simulink model "c221127_FCEV_SLMP_SQP"  (R2022b)
settings: Solver=FixedStepAuto  StartTime=0.0  StopTime=DrvCycLen  FixedStep=1  RelTol=1e-3
values from neighbouring files (symbols this model uses):
  AccThrshd = 1    [Config_c221112.m]    (also in Config_c221127.m; Config_c221218.m; Config_c230117.m; Config_c230321.m)
  AlphaRampFactor = 8    [Config_c221112.m]    (also in Config_c221127.m; Config_c221218.m; Config_c230117.m; Config_c230321.m)
  Bat_eff_chg_average = 0.969    [FCEV_original_data.mat]
  Bat_eff_dis_average = 0.9632    [FCEV_original_data.mat]
  Bat_end_of_life_percent = 20    [FCEV_original_data.mat]
  Bat_I_chg_max = -120    [FCEV_original_data.mat]
  Bat_I_dis_max = 200    [FCEV_original_data.mat]
  Bat_nom_Ic = 2.5    [FCEV_original_data.mat]
  Bat_nom_SOC = 0.35    [FCEV_original_data.mat]
  Bat_nom_temp_oC = 25    [FCEV_original_data.mat]
  Bat_num_pa = 9    [FCEV_original_data.mat]
  Bat_num_se = 97    [FCEV_original_data.mat]
  Bat_ori_C1_chg_F = [397.526659684 455.660832136 435.08783522 460.845064365 457.605812374 417.289828504 416.373906992 359.741413056 321.561704819 1109.14132554 1165.67733205 1135.97600211 ... (72 elements, 9x8)]    [FCEV_original_data.mat]
  Bat_ori_C1_dis_F = [187.121968588 287.083505726 346.448009002 395.529439835 387.517274826 389.973134196 432.856765051 486.92921923 512.158935268 425.990733989 614.68708868 771.472592368 ... (72 elements, 9x8)]    [FCEV_original_data.mat]
  Bat_ori_C2_chg_F = [8748.48589695 7773.35875681 9404.86567646 8934.73981058 8290.58671366 7592.78422269 7759.44623103 7396.59043829 6151.35152293 16187.7227039 11721.8480541 13157.8579836 ... (72 elements, 9x8)]    [FCEV_original_data.mat]
  Bat_ori_C2_dis_F = [2939.81325553 4590.73311898 5504.93546413 5887.5077374 6534.37836712 7765.46899768 10584.7751706 10372.0508438 9238.72693885 5207.86390693 7911.43744944 8879.62137571 ... (72 elements, 9x8)]    [FCEV_original_data.mat]
  Bat_ori_cap_max_Ah = 20.7    [Config_c221218.m]    (also in Config_c230117.m; Config_c230321.m; FCEV_original_data.mat)
  Bat_ori_dUdt4 = [-0.303773584906 -0.249056603774 -0.115094339623 -0.0396226415094 0.0396226415094 0.0641509433962 0.107547169811 0.111320754717 0.0415094339623 0.0547169811321 0.130188679245]    [FCEV_original_data.mat]
  Bat_ori_R0_chg_O = [0.0771669453735 0.0731809311402 0.0726556782939 0.0729965156794 0.0731758310684 0.0742031005051 0.0721266921026 0.0714211058078 0.0714186176143 0.0374124505155 0.0354566732504 0.0345430657188 ... (72 elements, 9x8)]    [FCEV_original_data.mat]
  Bat_ori_R0_dis_O = [0.0819458671157 0.0812429476608 0.0803749674507 0.0805513601722 0.0838629023857 0.0850797840015 0.0829875518672 0.0826388888889 0.0812514106148 0.0428124986417 0.0424658903711 0.0428572670451 ... (72 elements, 9x8)]    [FCEV_original_data.mat]
  Bat_ori_R1_chg_O = [0.114339870884 0.105392753268 0.104421193553 0.109821896183 0.114868279838 0.123333154908 0.129174812826 0.149917249373 0.174896487845 0.0420560161846 0.0390948352938 0.0370122837364 ... (72 elements, 9x8)]    [FCEV_original_data.mat]
  Bat_ori_R1_dis_O = [0.304806399643 0.213604089624 0.171463520004 0.151183840498 0.140630862434 0.128795299077 0.116857791733 0.112567113582 0.106368362501 0.0943235089866 0.0730697254134 0.0611414736086 ... (72 elements, 9x8)]    [FCEV_original_data.mat]
  Bat_ori_R2_chg_O = [0.134518959939 0.17565045702 0.161100627268 0.189032232545 0.205639040497 0.226170473035 0.223651875822 0.181765694192 0.212966950836 0.073628872144 0.0788540822416 0.0792414571734 ... (72 elements, 9x8)]    [FCEV_original_data.mat]
  Bat_ori_R2_dis_O = [0.354968099904 0.285293035102 0.286338708953 0.298763853987 0.248762838155 0.178586175471 0.129047399775 0.188406991173 0.174494800676 0.131839238891 0.123225430215 0.132069033134 ... (72 elements, 9x8)]    [FCEV_original_data.mat]
  Bat_ori_SOC2 = [0 0.001 0.002 0.003 0.004 0.005 0.006 0.007 0.008 0.009 0.01 0.011 ... (1001 elements, 1x1001)]    [FCEV_original_data.mat]
  Bat_ori_SOC4 = [-0.00598301069999 0.0920117618231 0.190864167279 0.289083557951 0.387343788287 0.485011843502 0.5850485992 0.678163031937 0.774810095565 0.876684636119 0.972739524626]    [FCEV_original_data.mat]
  Bat_ori_Uoc_chg_V = [2.4478 2.54923264342 2.6007 2.6383 2.66953057366 2.69636321708 2.7197 2.74042850391 2.75906114733 2.77619379074 2.792 2.80675907757 ... (1001 elements, 1x1001)]    [FCEV_original_data.mat]
  Bat_ori_Uoc_dis_V = [1.9998 2.03916768329 2.24724374236 2.39700902919 2.48767431602 2.5476 2.5882 2.6202 2.64771773167 2.6719 2.6933 2.71251566192 ... (1001 elements, 1x1001)]    [FCEV_original_data.mat]
  Bat_ori_Uoc_V = [2.2238 2.29420016335 2.42397187118 2.5176545146 2.57860244484 2.62198160854 2.65395 2.68031425195 2.7033894395 2.72404689537 2.74265 2.75963736975 ... (1001 elements, 1x1001)]    [FCEV_original_data.mat]
  Bat_power_max_kW = 50    [FCEV_original_data.mat]
  Bat_power_min_kW = 0    [FCEV_original_data.mat]
  Bat_single_capacity_nom_Ah = 2.3    [FCEV_original_data.mat]
  Bat_SOC_ini = 0.3    [Config_c22100601.m]    (also in Config_c22100701.m; FCEV_original_data.mat = 0.45)
  Bat_SOC_max = 0.9    [FCEV_original_data.mat]
  Bat_SOC_min = 0.3    [FCEV_original_data.mat]
  Bat_temp_amb_oC = 25    [FCEV_original_data.mat]
  Bat_temp_cool_oC = 25    [FCEV_original_data.mat]
  BattInitTemp = 25    [Config_c221127.m]    (also in Config_c221218.m; Config_c230117.m; Config_c230321.m)
  BattOnly = 0    [Config_c221218.m]    (also in Config_c230117.m = BattSocRightNow > BattSocLowerLimit; Config_c230321.m = double(BattSocRightNow > BattSocLowerLimit))
  BattSocInit = 0.9    [Config_c221112.m]    (also in Config_c221127.m = 0.3; Config_c221218.m = 0.3; Config_c230117.m = 0.8; Config_c230321.m = 0.8)
  BattSocLowerLimit = 0.25    [Config_c221112.m]    (also in Config_c221127.m = 0.3; Config_c221218.m = 0.3; Config_c230117.m = 0.3; Config_c230321.m = 0.3)
  BattSocRightNow = BattSocRightNow - SocDrop    [Config_c221218.m]    (also in Config_c230117.m; Config_c230321.m)
  BattSocUpperLimit = 0.9    [Config_c221112.m]    (also in Config_c221127.m = 0.8; Config_c221218.m = 0.8; Config_c230117.m = 0.8; Config_c230321.m = 0.8)
  CFWF = 0.5    [Config_c221127.m]    (also in Config_c221218.m; Config_c230117.m; Config_c230321.m)
  DCAC_eff = 0.95    [FCEV_original_data.mat]
  DCDC_ori_eff = [0.95 0.96 0.97 0.976 0.98 0.978 0.973 0.962]    [FCEV_original_data.mat]
  DCDC_ori_power_kW = [0 10 20 30 40 50 60 70]    [FCEV_original_data.mat]
  DeAccThrshd = -1    [Config_c221112.m]    (also in Config_c221127.m; Config_c221218.m; Config_c230117.m; Config_c230321.m)
  DeltaFcPwrRcm_down = 0.5    [Config_c221127.m]    (also in Config_c221218.m; Config_c230117.m; Config_c230321.m)
  DeltaFcPwrRcm_up = 2    [Config_c221127.m]    (also in Config_c221218.m = 3; Config_c230117.m = 4; Config_c230321.m = 4)
  DrvCycRange = sum(DrvCycVps(:,2))    [Config_c221112.m]    (also in Config_c221127.m; Config_c221218.m; Config_c230117.m; Config_c230321.m)
  FC_ori_eff = [0.1 0.33 0.492 0.533 0.559 0.596 0.591 0.562 0.508]    [FCEV_original_data.mat]
  FC_ori_fuel_rate_gps = [0 0.0505050505051 0.0846883468835 0.117260787992 0.149075730471 0.279642058166 0.423011844332 0.593119810202 0.820209973753]    [FCEV_original_data.mat]
  FC_ori_power_kW = [0 2 5 7.5 10 20 30 40 50]    [FCEV_original_data.mat]
  FC_power_max_kW = 50    [FCEV_original_data.mat]
  FC_power_min_kW = 0    [FCEV_original_data.mat]
  FcPwrDropCall = 6    [Config_c221127.m]    (also in Config_c221218.m; Config_c230117.m; Config_c230321.m)
  HydpriceRmb = 30    [Config_c221127.m]    (also in Config_c221218.m; Config_c230117.m; Config_c230321.m)
  m = Time_sample    [Config_c22100601.m]    (also in Config_c22100701.m)
  MC_eff_brk_average = 0.810578512397    [FCEV_original_data.mat]
  MC_eff_dri_average = 0.810578512397    [FCEV_original_data.mat]
  MC_inertia = 0.06    [FCEV_original_data.mat]
  MC_ori_eff = [0.7 0.78 0.85 0.86 0.81 0.82 0.79 0.78 0.78 0.78 0.78 0.7 ... (231 elements, 11x21)]    [FCEV_original_data.mat]
  MC_ori_power_brk_req_kW = [0 -28.3912930389 -56.7825860779 -85.1738791168 -113.565172156 -141.956465195 -170.347758234 -198.739051273 -227.130344311 -255.52163735 -283.912930389 0 ... (121 elements, 11x11)]    [FCEV_original_data.mat]
  MC_ori_power_dri_req_kW = [0 0 0 0 0 0 0 0 0 0 0 0 ... (121 elements, 11x11)]    [FCEV_original_data.mat]
  MC_ori_spd_rpm = [0 1000 2000 3000 4000 5000 6000 7000 8000 9000 10000]    [FCEV_original_data.mat]
  MC_ori_trq_brk_max_Nm = [-271.1368 -271.1368 -271.1368 -237.5159 -178.1369 -142.4824 -118.7579 -101.8119 -89.0685 -79.172 -71.1734]    [FCEV_original_data.mat]
  MC_ori_trq_brk_Nm = [-271.136848522 -244.02316367 -216.909478817 -189.795793965 -162.682109113 -135.568424261 -108.454739409 -81.3410545565 -54.2273697044 -27.1136848522 0]    [FCEV_original_data.mat]
  MC_ori_trq_dri_max_Nm = [271.1368 271.1368 271.1368 237.5159 178.1369 142.4824 118.7579 101.8119 89.0685 79.172 71.1734]    [FCEV_original_data.mat]
  MC_ori_trq_dri_Nm = [0 27.1136848522 54.2273697044 81.3410545565 108.454739409 135.568424261 162.682109113 189.795793965 216.909478817 244.02316367 271.136848522]    [FCEV_original_data.mat]
  MC_ori_trq_Nm = [-271.136848522 -244.02316367 -216.909478817 -189.795793965 -162.682109113 -135.568424261 -108.454739409 -81.3410545565 -54.2273697044 -27.1136848522 0 27.1136848522 ... (21 elements, 1x21)]    [FCEV_original_data.mat]
  MC_power_max_kW = 75    [FCEV_original_data.mat]
  MC_spd_max_rpm = 10000    [FCEV_original_data.mat]
  MC_spd_min_rpm = 0    [FCEV_original_data.mat]
  MC_spd_scale = 1    [FCEV_original_data.mat]
  MC_trq_scale = 1    [FCEV_original_data.mat]
  MC_U_min_V = 120    [FCEV_original_data.mat]
  no_FcPwrSlowDrop = 1    [Config_c230321.m]
  Placeholder = 0    [Config_c221127.m]    (also in Config_c221218.m; Config_c230117.m; Config_c230321.m)
  PredLen = 5    [Config_c221112.m]    (also in Config_c221127.m; Config_c221218.m; Config_c230117.m; Config_c230321.m)
  Road_u = 0.75    [FCEV_original_data.mat]
  SC_np = 1    [Config_c230321.m]
  SC_ns = 100    [Config_c230321.m]
  SC_rc = 1000    [Config_c230321.m]
  SLMP_LearningRate = 0.05    [Config_c221112.m]    (also in Config_c221127.m; Config_c221218.m; Config_c230117.m; Config_c230321.m)
  tDegTable = [zeros(1,3),linspace(0,0.13,47)]    [Config_c221127.m]    (also in Config_c221218.m; Config_c230117.m; Config_c230321.m)
  usd2rmb = 7.116    [Config_c22100601.m]    (also in Config_c22100701.m; Config_c221106.m = 6; Config_c221112.m = 6; Config_c221127.m = 6)
  Veh_air_density_kgpm2 = 1.2    [FCEV_original_data.mat]
  Veh_brk_front = [1 0.6 0.608 0.61 0.618 0.624 0.636 0.645 0.655]    [FCEV_original_data.mat]
  Veh_brk_z = [0.1 0.2 0.3 0.4 0.5 0.6 0.7 0.8 0.9]    [FCEV_original_data.mat]
  Veh_brk_z_max = 0.7    [FCEV_original_data.mat]
  Veh_brk_z_min = 0.1    [FCEV_original_data.mat]
  Veh_coeff_drag = 0.312    [FCEV_original_data.mat]
  Veh_coeff_roll = 0.00863    [FCEV_original_data.mat]
  Veh_final_drive_inertia = 0.1105    [FCEV_original_data.mat]
  Veh_final_drive_ratio = 3.47    [FCEV_original_data.mat]
  Veh_frontal_area_m2 = 2.06    [FCEV_original_data.mat]
  Veh_gravity_acc_ms2 = 9.81    [FCEV_original_data.mat]
  Veh_mass_cargo_kg = 113    [FCEV_original_data.mat]
  Veh_mass_curb_kg = 1157    [FCEV_original_data.mat]
  Veh_mech_eff = 0.9    [FCEV_original_data.mat]
  Veh_rotary_mass_conversion_factor = 1.05    [FCEV_original_data.mat]
  Veh_size_cg_height_m = 0.53    [FCEV_original_data.mat]
  Veh_wheel_inertia = 3.1039    [FCEV_original_data.mat]
  Veh_wheel_radius_m = 0.313    [FCEV_original_data.mat]
  Veh_wt_frac_front = 0.5    [FCEV_original_data.mat]
  VstdThrshd = 2    [Config_c221112.m]    (also in Config_c221127.m; Config_c221218.m; Config_c230117.m; Config_c230321.m)
undefined symbols (not defined in the file or in its folder): Bat_ori_temp, SC_iv, SC_nm, SC_SocTable
libraries: autolibshared x2
(part 1 of 8)
settings Model: Creator=xuupp  LastModifiedBy=xuupp
settings DataIOCC: ReturnWorkspaceOutputs=off
settings RTWCC: GenCodeOnly=on

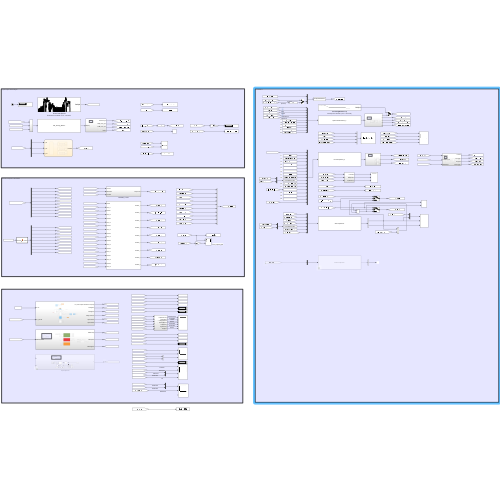
[thumbnail: Simulink's stored preview of the top-level diagram]
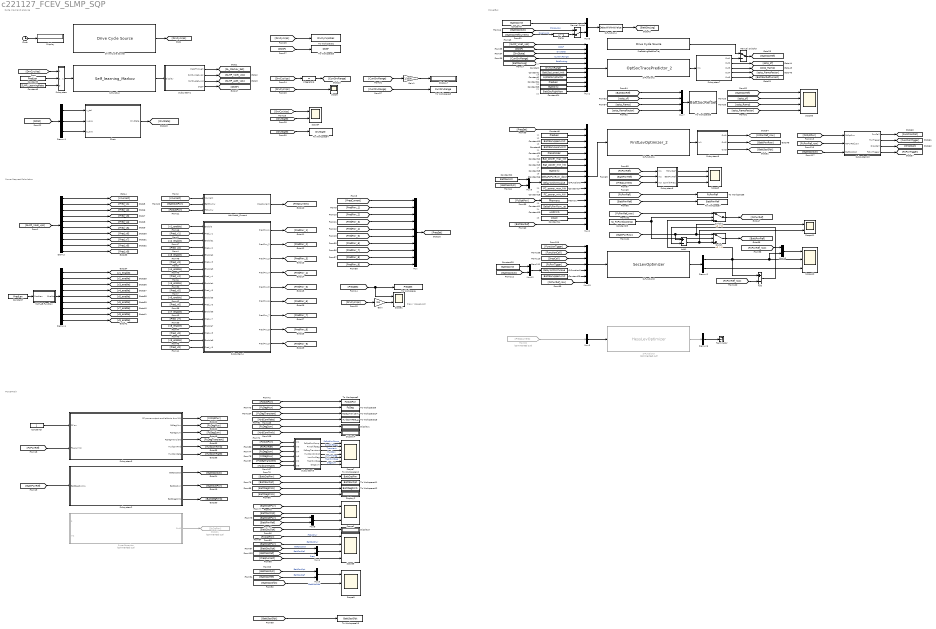
== system c221127_FCEV_SLMP_SQP ==
  note: 11
  note: PowerTrain
  note: Preq / Vspeed_kph
  note: PowerBus
  note: Power Request Calculation
  note: Cycle input and analyse
  note: 12
  note: 13
  note: 15
  note: 16
  note: 17
  note: 18
  note: 20
  note: 21
  note: 23
  note: 24
  note: 25
  note: 17
  note: 18
  note: 19
  note: 20
  note: 14
  note: 21
  note: 22
  Add : Sum  Inputs=+-
  Add1 : Sum  Inputs=+-
  Chart : Stateflow chart  TreatAsAtomicUnit=on
  Clock : Clock
  Constant : Constant  Value=DrvCycRange
  Constant1 : Constant  Value=BattSocLowerLimit
  Constant10 : Constant  Value=BattSocUpperLimit
  Constant11 : Constant  Value=DeltaFcPwrRcm_up
  Constant12 : Constant  Value=Bat_power_max_kW
  Constant13 : Constant  Value=Bat_power_min_kW
  Constant14 : Constant  Value=CFWF
  Constant15 : Constant  Value=BattOnly
  Constant16 : Constant  Value=DeltaFcPwrRcm_down
  Constant17 : Constant  Value=FC_power_max_kW
  Constant18 : Constant  Value=FC_power_min_kW
  Constant19 : Constant  Value=usd2rmb
  Constant2 : Constant  Value=AlphaRampFactor
  Constant20 : Constant  Value=Placeholder
  Constant{5,7..8,21} (4 alike) : Constant  Value=PredLen
  Constant22 : Constant  Value=BattSocInit
  Constant23 : Constant  Value=BattOnly
  Constant24 : Constant  Value=BattSocRightNow
  Constant25 : Constant  Value=no_FcPwrSlowDrop
  Constant28 : Constant  Value=BattSocInit
  Constant29 : Constant  Value=BattSocUpperLimit
  Constant3 : Constant
  Constant4 : Constant  Value=BattSocInit
  Constant6 : Constant  Value=SLMP_LearningRate
  Constant9 : Constant  Value=BattSocLowerLimit
  Delay : Delay  DelayLength=1
  Demux : Demux  Outputs=10
  Demux1 : Demux  Outputs=3
  Demux2 : Demux  Outputs=2
  Demux4 : Demux  Outputs=9
  Demux6 : Demux  Outputs=1
  Display{,1..4,7} (6 alike) : Display
  Drive Cycle Source : autolibshared/Drive Cycle Source  cycleVar=Workspace variable  wsVar=DrvCycVps  fileVar=cycleFTP75.mat  tfinal="7031  seconds"  cycleRepeat=off  outAccPort=off  outGearPort=off  gearList=No gear data  t_wot1=5  xdot_woto=0  xdot_wot1=30  t_wot2=20  xdot_wot2=0  t_wotend=30  srcUnit=m/s  outUnit=m/s  srcAccUnit=m/s/s  outAccUnit=m/s^2  dt=1  aMode=1  faultOption=off  velBnd=2  velBndUnit=mph  inUnit=m/s  timeBnd=1  failOption=off  stopSim=off  maxFaultCnt=10  maxFaultTime=2  maxTotFaultTime=15  traceOption=off  dtTrace=1  traceWindow=10  lastDCname=Custom Data Set  lastOutUnit=mph  lastDT=1  lastTB=1  lastSB=2  forceCalcBound=off
  From32 : From  Commented=on  GotoTag=PreqCurrent
  Gain : Gain  Gain=3.6
  Gain1 : Gain  Gain=1/1000
  Goto21 : Goto  Commented=on  GotoTag=ScOpPwr
  Integrator6 : Integrator
  MATLAB Function : MATLAB Function  TreatAsAtomicUnit=on
  Manual Switch : ManualSwitch  CurrentSetting=0
  Manual Switch3 : ManualSwitch
  Memory : Memory
  Mux : Mux  Inputs=10
  Mux1 : Mux  Inputs=11
  Mux{4..6,8..10,12} (7 alike) : Mux  Inputs=2
  Mux13 : Mux  Inputs=7
  Mux2 : Mux  Inputs=17
  Mux3 : Mux  Inputs=1
  Mux7 : Mux
  PreSettingBattSocTraj : autolibshared/Drive Cycle Source  cycleVar=Workspace variable  wsVar=tbSoc_ref  fileVar=cycleFTP75.mat  tfinal="7031  seconds"  cycleRepeat=off  outAccPort=off  outGearPort=off  gearList=No gear data  t_wot1=5  xdot_woto=0  xdot_wot1=30  t_wot2=20  xdot_wot2=0  t_wotend=30  srcUnit=m/s  outUnit=m/s  srcAccUnit=m/s/s  outAccUnit=m/s^2  dt=1  aMode=1  faultOption=off  velBnd=2  velBndUnit=mph  inUnit=m/s  timeBnd=1  failOption=off  stopSim=off  maxFaultCnt=10  maxFaultTime=2  maxTotFaultTime=15  traceOption=off  dtTrace=1  traceWindow=10  lastDCname=Custom Data Set  lastOutUnit=mph  lastDT=1  lastTB=1  lastSB=2  forceCalcBound=off
  S-Function : S-Function  FunctionName=Self_learning_Markov  SFunctionDeploymentMode=off  EnableBusSupport=off
  S-Function1 : S-Function  FunctionName=FirstLevOptimizer_2  SFunctionDeploymentMode=off  EnableBusSupport=off
  S-Function2 : S-Function  FunctionName=OptSocTracePredictor_2  SFunctionDeploymentMode=off  EnableBusSupport=off
  S-Function3 : S-Function  Commented=on  FunctionName=HessLevOptimizer  SFunctionDeploymentMode=off  EnableBusSupport=off
  S-Function4 : S-Function  FunctionName=DelayWithInitValue  SFunctionDeploymentMode=off  EnableBusSupport=off
  S-Function5 : S-Function  FunctionName=DelayWithInitValue  SFunctionDeploymentMode=off  EnableBusSupport=off
  S-Function8 : S-Function  FunctionName=SecLevOptimizer  SFunctionDeploymentMode=off  EnableBusSupport=off
  S-Function9 : S-Function  FunctionName=DelayWithInitValue  SFunctionDeploymentMode=off  EnableBusSupport=off
  Scope : Scope
  Scope1 : Scope  NumInputPorts=2
  Scope{2,5,9..10} (4 alike) : Scope  NumInputPorts=3
  Scope11 : Scope  NumInputPorts=2
  Scope4 : Scope  NumInputPorts=2
  Scope6 : Scope  NumInputPorts=4
  Scope7 : Scope  NumInputPorts=7
  Scope8 : Scope  NumInputPorts=4
  Subsystem : Subsystem
  Subsystem1 : Subsystem
  Subsystem10 : Subsystem
  Subsystem2 : Subsystem
  Subsystem3 : Subsystem
  Subsystem4 : Subsystem
  Subsystem5 : Subsystem
  Subsystem6 : Subsystem
  Subsystem7 : Subsystem
  Subsystem8 : Subsystem
  SuperCapacitor : Subsystem  Commented=on
  Switch : Switch  Criteria=u2 > Threshold  SaturateOnIntegerOverflow=off  InputSameDT=off
  Switch1 : Switch  Criteria=u2 > Threshold  SaturateOnIntegerOverflow=off  InputSameDT=off
  Terminator : Terminator
  To Workspace : ToWorkspace  VariableName=PreqSet  SampleTime=-1
  To Workspace1 : ToWorkspace  VariableName=DrvCycVpsRec  SampleTime=-1
  To Workspace10 : ToWorkspace  VariableName=BattOptPwr  SampleTime=-1
  To Workspace11 : ToWorkspace  VariableName=BattSocOpt  SampleTime=-1
  To Workspace12 : ToWorkspace  VariableName=BattDegRmb  SampleTime=-1
  To Workspace13 : ToWorkspace  VariableName=BattSocOfst  SampleTime=-1
  To Workspace14 : ToWorkspace  VariableName=FcDegTranisent  SampleTime=-1
  To Workspace15 : ToWorkspace  VariableName=HydComRate_g  SampleTime=-1
  To Workspace2 : ToWorkspace  VariableName=FcOptPwr  SampleTime=-1
  To Workspace3 : ToWorkspace  VariableName=DCSF  SampleTime=-1
  To Workspace4 : ToWorkspace  VariableName=DrvState  SampleTime=-1
  To Workspace5 : ToWorkspace  VariableName=CurrDrvRange  SampleTime=-1
  To Workspace6 : ToWorkspace  VariableName=FcPwrRef  SampleTime=-1
  To Workspace7 : ToWorkspace  VariableName=BattPwrRef  SampleTime=-1
  To Workspace8 : ToWorkspace  VariableName=BattSocRefSet  SampleTime=-1
  To Workspace9 : ToWorkspace  VariableName=FcDeg  SampleTime=-1
  VehModel_Current : Subsystem
  wires:
  S-Function/1 -> Subsystem1/1(Display)
  [DrvCycVps] -> Subsystem/1(RowSequence)
  Drive Cycle Source/1 -> [DrvCycVps]
  Clock/1 -> Display/1
  Subsystem1/3(SLMP_aset_vps) -> [SLMP_aset_vps]
  Subsystem/1(HstLog) -> S-Function/1
  Subsystem1/1(PassThrough) -> [SL_Markov_Set]
  Subsystem1/2(SLMP_Vset_vps) -> [SLMP_Vset_vps]
  [SLMP_Vset_vps] -> Demux/1
  Demux/1 -> [Vcurrent]
  Demux/2 -> [Pred_v1]
  Demux/3 -> [Pred_v2]
  Demux/4 -> [Pred_v3]
  Demux/5 -> [Pred_v4]
  Demux/6 -> [Pred_v5]
  [Vcurrent] -> VehModel_Current/1(Vcurrent)
  VehModel_Current/1(PreqCurrent) -> [PreqCurrent]
  [PreqCurrent] -> Mux/1
  [PredPwr_1] -> Mux/2
  [PredPwr_2] -> Mux/3
  [PredPwr_3] -> Mux/4
  [PredPwr_4] -> Mux/5
  [PredPwr_5] -> Mux/6
  Mux/1 -> [PreqSet]
  [DCSF] -> Demux1/1
  [DrvCycVps] -> Scope/1
  [DrvCycVps] -> Integrator6/1
  [DrvCycVps] -> To Workspace1/1
  Subsystem1/4(DCSF) -> [DCSF]
  [DCSF] -> To Workspace3/1
  Demux1/1 -> Chart/1(v_std)
  Demux1/2 -> Chart/2(v_ave)
  Demux1/3 -> Chart/3(a_ave)
  Chart/1(DrvState) -> [DrvState]
  [DrvCycVps] -> Scope4/1
  [DrvState] -> Scope4/2
  [DrvState] -> To Workspace4/1
  Subsystem3/1(FC power output avaliable to bus (kW)) -> [FcOptPwr]
  SuperCapacitor/1(Out1) -> Goto21/1
  Subsystem3/2(FcDegMux) -> [FcDegMux]
  Mux2/1 -> S-Function1/1
  From32/1 -> Mux3/1
  Integrator6/1 -> [CurrDrvRange]
  [CurrDrvRange] -> Gain1/1
  Subsystem2/2(BattOpPwr) -> [BattOptPwr]
  Subsystem2/1(BattSocOpt) -> [BattSocOpt]
  Mux1/1 -> S-Function2/1
  Constant2/1 -> Mux1/8
  Constant1/1 -> Mux1/7
  [CurrDrvRange] -> Mux1/4  "CurrDrvRange"
  [DCSF] -> Mux1/2  "DCSF"
  Constant/1 -> Mux1/6
  [DrvState] -> Mux1/3  "DrvState"
  [CurrDrvRange] -> To Workspace5/1
  Constant5/1 -> Subsystem/2(RowSequence1)
  Constant6/1 -> Subsystem/3(RowSequence2)
  Demux/7 -> [Pred_v6]
  Demux/8 -> [Pred_v7]
  Demux/9 -> [Pred_v8]
  Demux/10 -> [Pred_v9]
  Constant7/1 -> MATLAB Function/1(PredLen)
  MATLAB Function/1(Enable) -> Demux4/1
  Demux4/1 -> [v1_enable]
  Demux4/2 -> [v2_enable]
  Demux4/3 -> [v3_enable]
  Demux4/4 -> [v4_enable]
  Demux4/5 -> [v5_enable]
  Demux4/6 -> [v6_enable]
  Demux4/7 -> [v7_enable]
  Demux4/8 -> [v8_enable]
  Demux4/9 -> [v9_enable]
  [v1_enable] -> Subsystem4/1(Enable)
  [Pred_v1] -> Subsystem4/2(Pred_v1)
  [v2_enable] -> Subsystem4/3(Enable1)
  [Pred_v2] -> Subsystem4/4(Pred_v2)
  [v3_enable] -> Subsystem4/5(Enable2)
  [Pred_v3] -> Subsystem4/6(Pred_v3)
  [v4_enable] -> Subsystem4/7(Enable3)
  [Pred_v4] -> Subsystem4/8(Pred_v4)
  [v5_enable] -> Subsystem4/9(Enable4)
  [Pred_v5] -> Subsystem4/10(Pred_v5)
  [v6_enable] -> Subsystem4/11(Enable5)
  [Pred_v6] -> Subsystem4/12(Pred_v6)
  [v7_enable] -> Subsystem4/13(Enable6)
  [Pred_v7] -> Subsystem4/14(Pred_v7)
  [v8_enable] -> Subsystem4/15(Enable7)
  [Pred_v8] -> Subsystem4/16(Pred_v8)
  [v9_enable] -> Subsystem4/17(Enable8)
  [Pred_v9] -> Subsystem4/18(Pred_v9)
  Subsystem4/1(PredPwr_1) -> [PredPwr_1]
  Subsystem4/2(PredPwr_2) -> [PredPwr_2]
  Subsystem4/3(PredPwr_3) -> [PredPwr_3]
  Subsystem4/4(PredPwr_4) -> [PredPwr_4]
  Subsystem4/5(PredPwr_5) -> [PredPwr_5]
  Subsystem4/6(PredPwr_6) -> [PredPwr_6]
  Subsystem4/7(PredPwr_7) -> [PredPwr_7]
  Subsystem4/8(PredPwr_8) -> [PredPwr_8]
  Subsystem4/9(PredPwr_9) -> [PredPwr_9]
  [PredPwr_6] -> Mux/7
  [PredPwr_7] -> Mux/8
  [PredPwr_8] -> Mux/9
  [PredPwr_9] -> Mux/10
  [PreqSet] -> Mux2/1
  Constant8/1 -> Mux2/2
  Constant10/1 -> Mux2/3
  Constant9/1 -> Mux2/4
  Constant20/1 -> Mux2/5
  Constant12/1 -> Mux2/6
  Constant13/1 -> Mux2/7
  Constant16/1 -> Mux2/9
  Constant17/1 -> Mux2/11
  Constant18/1 -> Mux2/12
  [FcOptPwr] -> Memory/1
  [PreqSet] -> Scope1/1, To Workspace/1
  [DrvCycVps] -> Gain/1
  Gain/1 -> Scope1/2
  Constant11/1 -> Mux2/14
  Constant14/1 -> Mux2/16
  [BattSocLog] -> Mux1/5  "BattSocLog"
  Mux3/1 -> S-Function3/1
  S-Function3/1 -> Demux6/1
  Demux6/1 -> Terminator/1
  [FcPwrRef] -> Subsystem3/2("FC_pwr kW ")
  [BattPwrRef] -> Subsystem2/1(BattReqPwrKw)
  Constant3/1 -> Subsystem3/1(FC on)
  [BattSocRef] -> Scope6/1
  [ostp_sf] -> Scope6/2
  [ostp_Ramp] -> Scope6/3
  [ostp_RampFactor] -> Scope6/4
  [BattSocRef] -> Mux7/1
  [ostp_sf] -> Mux7/2
  [ostp_Ramp] -> Mux7/3
  [ostp_RampFactor] -> Mux7/4
  [FcPwrRef] -> To Workspace6/1
  [BattPwrRef] -> To Workspace7/1
  [FcPwrRef] -> Subsystem6/1(In1)
  [BattPwrRef] -> Subsystem6/2(In2)
  Constant19/1 -> Mux2/15
  S-Function4/1 -> [BattSocLog]
  Mux6/1 -> S-Function4/1
  [BattSocOpt] -> Manual Switch/1  "CloseLoop"
  Constant4/1 -> Mux6/1
  [BattOptPwr] -> VehModel_Current/2(BattPwrKw)
  [FcOptPwr] -> VehModel_Current/3(FcPwrKw)
  Mux7/1 -> To Workspace8/1
  [FcDegMux] -> To Workspace9/1
  [BattOptPwr] -> To Workspace10/1
  [BattSocOpt] -> To Workspace11/1
  [FcOptPwr] -> To Workspace2/1
  [BattPwrRef] -> Mux8/2
  [BattOptPwr] -> Mux8/1
  [BattSocOpt] -> Scope2/2
  [BattOptPwr] -> Scope2/1
  Mux8/1 -> Scope2/3
  Subsystem3/3(FcDegSum) -> [FcDegSum]
  [FcOptPwr] -> Scope8/1  "FcOptPwr"
  [BattOptPwr] -> Scope8/2  "BattOptPwr"
  [FcOptPwr] -> Subsystem5/1(In1)
  [FcDegSum] -> Subsystem5/3(In4)
  [FcDegMux] -> Subsystem5/4(In5)
  Subsystem5/1(FcOptPwrComp) -> Scope7/1  "FcOptPwrComp"
  Subsystem5/2(PwrShiftDeg) -> Scope7/2  "PwrShiftDeg"
  Subsystem5/3(FcDegTransient) -> Scope7/3  "Transient"
  Subsystem5/5(LowPwrDeg) -> Scope7/5  "LowPwrDeg"
  Subsystem5/6(HighPwrDeg) -> Scope7/6  "HighPwrDeg"
  [FcPwrRef] -> Subsystem5/2(In3)
  [FcDegSum] -> Display1/1
  Subsystem2/3(BattDegRmb) -> [BattDegRmb]
  [BattDegRmb] -> To Workspace12/1
  [BattDegRmb] -> Display2/1
  [PreqCurrent] -> Subsystem6/3(In3)
  Subsystem6/1(FcPwrRef) -> Scope5/1
  Subsystem6/2(BattPwrRef) -> Scope5/2
  Subsystem6/3(CprWithPreq) -> Scope5/3
  [BattSocOpt] -> Mux4/1  "BattSocOpt"
  [PreqCurrent] -> Scope8/4  "Preq"
  Memory/1 -> Mux2/13
  Gain1/1 -> Display7/1
  [SLMP_Vset_vps] -> Mux1/1
  Constant21/1 -> Mux1/9
  S-Function2/1 -> Subsystem7/1(In1)
  Subsystem7/1(Out1) -> Manual Switch3/2
  Subsystem7/2(Out2) -> [ostp_sf]
  Subsystem7/3(Out3) -> [ostp_Ramp]
  Subsystem7/4(Out4) -> [ostp_RampFactor]
  [BattSocRef] -> Mux2/17
  [BattSocRefCurrent] -> Delay/1  "OpenLoop"
  Manual Switch/1 -> Mux6/2
  Subsystem7/5(Out5) -> [BattSocRefCurrent]
  Mux4/1 -> Scope8/3
  [BattSocRef] -> Mux4/2  "BattSocRef"
  [BattSocOfst] -> Scope9/2  "BattSocOfst"
  [BattSocOpt] -> Mux5/1  "BattSocOpt"
  [BattSocRef] -> Mux5/2  "BattSocRef"
  Mux5/1 -> Scope9/1
  [BattSocOfst] -> To Workspace13/1
  S-Function5/1 -> Mux2/10
  Mux9/1 -> S-Function5/1
  [BattSocOpt] -> Mux9/2
  Constant22/1 -> Mux9/1
  S-Function1/1 -> Subsystem8/1(In1)
  Subsystem8/1(Out1) -> [FcPwrRef_row]
  Subsystem8/2(Out2) -> [BattPwrRow]
  Subsystem8/3(Out3) -> [BattSocOfst]
  [BattSocOpt] -> Display3/1
  Subsystem3/4(FcDegTransient) -> [FcDegTransient]
  [FcDegTransient] -> Subsystem5/5(In2)
  Subsystem5/7(DegSum) -> Scope7/7  "DegSum"
  [FcPwrRef_row] -> Switch1/1
  [FcDegTransient] -> To Workspace14/1
  Subsystem3/5(HydConRmb) -> [HydComRmb]
  [HydComRate] -> To Workspace15/1
  [HydComRmb] -> Display4/1
  Subsystem3/6(HydConRate) -> [HydComRate]
  [HydComRate] -> Subsystem5/6(In6)
  Subsystem5/4(HydConRmbIst) -> Scope7/4  "HydCon"
  Constant28/1 -> Mux12/1
  [BattSocOpt] -> Mux12/2
  Mux12/1 -> S-Function9/1
  [FunctionCall] -> Mux13/2
  [FunctionTigger] -> Mux13/1
  [DropCall] -> Mux13/3
  [FcPwrTigger] -> Mux13/4
  S-Function9/1 -> Mux13/5
  Constant29/1 -> Mux13/6
  Mux13/1 -> S-Function8/1
  [FcOptPwr] -> Subsystem10/1(FcOptPwr)
  [FcPwrRef_row] -> Subsystem10/2(FcPwrRef_row)
  [BattSocOpt] -> Subsystem10/3(BattSocOpt)
  Subsystem10/2(FunTigger) -> [FunctionTigger]
  Subsystem10/3(DropCall) -> [DropCall]
  Subsystem10/1(FunCall) -> [FunctionCall]
  S-Function8/1 -> Demux2/1
  Demux2/2 -> Scope10/3
  [FcPwrRef_row] -> Mux10/1
  Mux10/1 -> Scope10/1
  [FcPwrRef_row] -> Mux13/7
  Subsystem10/4(FcPwrTigger) -> [FcPwrTigger]
  Demux2/1 -> Switch1/3, Add/1, Scope10/2, Mux10/2
  [FcPwrRef_row] -> Add/2
  Add/1 -> Add1/2
  [BattPwrRow] -> Scope11/1, Switch/1, Add1/1
  Add1/1 -> Scope11/2, Switch/3
  Delay/1 -> Manual Switch/2
  Constant24/1 -> Mux1/11
  Constant23/1 -> Mux1/10
  PreSettingBattSocTraj/1 -> Manual Switch3/1
  Manual Switch3/1 -> [BattSocRef]
  Constant15/1 -> Mux2/8
  Switch/1 -> [BattPwrRef]
  Switch1/1 -> [FcPwrRef]
  Constant25/1 -> Switch/2, Switch1/2

== system c221127_FCEV_SLMP_SQP/Subsystem ==
  RowSequence : Inport
  RowSequence1 : Inport  Port=2
  RowSequence2 : Inport  Port=3
  Delay : Delay  DelayLength=1
  Delay1 : Delay
  Delay2 : Delay  DelayLength=3
  Delay3 : Delay  DelayLength=4
  Delay4 : Delay  DelayLength=5
  Delay5 : Delay  DelayLength=6
  Delay6 : Delay  DelayLength=7
  Delay7 : Delay  DelayLength=8
  Delay8 : Delay  DelayLength=9
  Mux : Mux  Inputs=12
  HstLog : Outport
  wires:
  RowSequence/1 -> Delay8/1, Delay7/1, Delay6/1, Delay5/1, Delay4/1, Delay3/1, Delay2/1, Delay1/1, Delay/1, Mux/1
  Mux/1 -> HstLog/1
  Delay8/1 -> Mux/10
  Delay7/1 -> Mux/9
  Delay6/1 -> Mux/8
  Delay5/1 -> Mux/7
  Delay3/1 -> Mux/5
  Delay2/1 -> Mux/4
  Delay1/1 -> Mux/3
  Delay/1 -> Mux/2
  Delay4/1 -> Mux/6
  RowSequence1/1 -> Mux/11
  RowSequence2/1 -> Mux/12

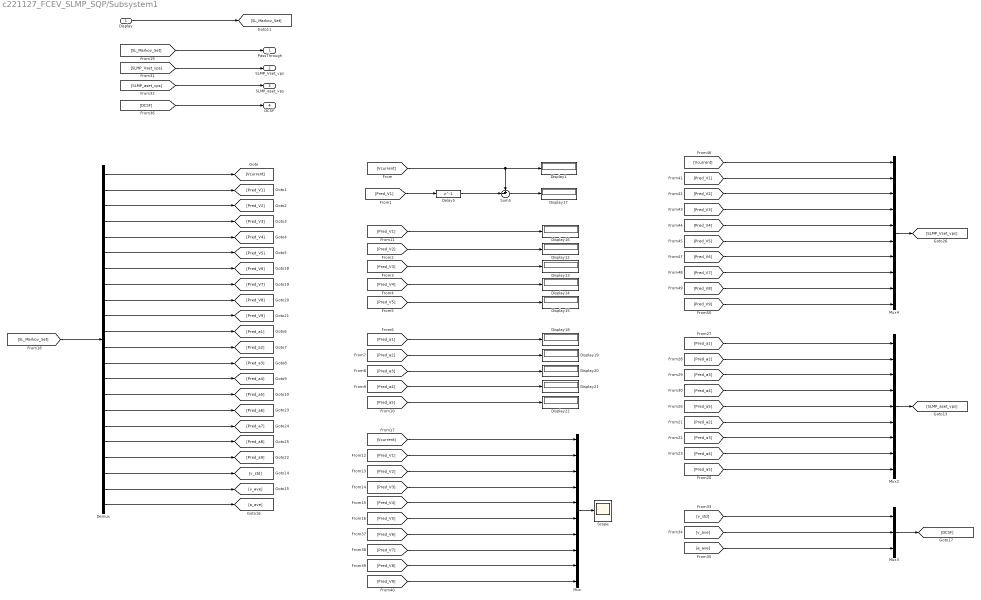
== system c221127_FCEV_SLMP_SQP/Subsystem1 ==
  Display : Inport
  Delay5 : Delay  DelayLength=1
  Demux : Demux  Outputs=22
  Display{1,12..22} (12 alike) : Display
  Mux : Mux  Inputs=10
  Mux2 : Mux  Inputs=9
  Mux3 : Mux  Inputs=3
  Mux4 : Mux  Inputs=10
  Scope : Scope
  Sum5 : Sum  Inputs=+-|
  PassThrough : Outport
  SLMP_Vset_vps : Outport  Port=2
  SLMP_aset_vps : Outport  Port=3
  DCSF : Outport  Port=4
  wires:
  Display/1 -> [SL_Markov_Set]
  Demux/1 -> [Vcurrent]
  Demux/2 -> [Pred_V1]
  Demux/3 -> [Pred_V2]
  Demux/4 -> [Pred_V3]
  Demux/5 -> [Pred_V4]
  Demux/6 -> [Pred_V5]
  [Pred_V1] -> Delay5/1
  Delay5/1 -> Sum5/2
  [Pred_V2] -> Display12/1
  [Pred_V3] -> Display13/1
  [Vcurrent] -> Display1/1, Sum5/1
  Sum5/1 -> Display17/1
  [Pred_V4] -> Display14/1
  [Pred_V5] -> Display15/1
  [Pred_V1] -> Display16/1
  [Pred_a1] -> Display18/1
  [Pred_a2] -> Display19/1
  [Pred_a3] -> Display20/1
  [Pred_a4] -> Display21/1
  [Pred_a5] -> Display22/1
  Mux/1 -> Scope/1
  [Pred_V5] -> Mux/6
  [Pred_V4] -> Mux/5
  [Pred_V3] -> Mux/4
  [Pred_V2] -> Mux/3
  [Pred_V1] -> Mux/2
  [Vcurrent] -> Mux/1
  [SL_Markov_Set] -> Demux/1
  [SL_Markov_Set] -> PassThrough/1
  [Pred_a3] -> Mux2/3
  [Pred_a2] -> Mux2/2
  [Pred_a1] -> Mux2/1
  [Pred_a4] -> Mux2/4
  [Pred_a5] -> Mux2/5
  Mux2/1 -> [SLMP_aset_vps]
  [SLMP_Vset_vps] -> SLMP_Vset_vps/1
  [SLMP_aset_vps] -> SLMP_aset_vps/1
  [v_std] -> Mux3/1
  [v_ave] -> Mux3/2
  [a_ave] -> Mux3/3
  Mux3/1 -> [DCSF]
  [DCSF] -> DCSF/1
  Demux/7 -> [Pred_V6]
  Demux/8 -> [Pred_V7]
  Demux/9 -> [Pred_V8]
  Demux/10 -> [Pred_V9]
  Demux/11 -> [Pred_a1]
  Demux/12 -> [Pred_a2]
  Demux/13 -> [Pred_a3]
  Demux/14 -> [Pred_a4]
  Demux/15 -> [Pred_a5]
  Demux/16 -> [Pred_a6]
  Demux/17 -> [Pred_a7]
  Demux/18 -> [Pred_a8]
  Demux/19 -> [Pred_a9]
  Demux/20 -> [v_std]
  Demux/21 -> [v_ave]
  Demux/22 -> [a_ave]
  [Pred_V6] -> Mux/7
  [Pred_V9] -> Mux/10
  [Pred_V7] -> Mux/8
  [Pred_V8] -> Mux/9
  [Pred_V8] -> Mux4/9
  [Pred_V7] -> Mux4/8
  [Pred_V9] -> Mux4/10
  [Pred_V6] -> Mux4/7
  [Vcurrent] -> Mux4/1
  [Pred_V1] -> Mux4/2
  [Pred_V2] -> Mux4/3
  [Pred_V3] -> Mux4/4
  [Pred_V4] -> Mux4/5
  [Pred_V5] -> Mux4/6
  Mux4/1 -> [SLMP_Vset_vps]
  [Pred_a2] -> Mux2/6
  [Pred_a3] -> Mux2/7
  [Pred_a4] -> Mux2/8
  [Pred_a5] -> Mux2/9

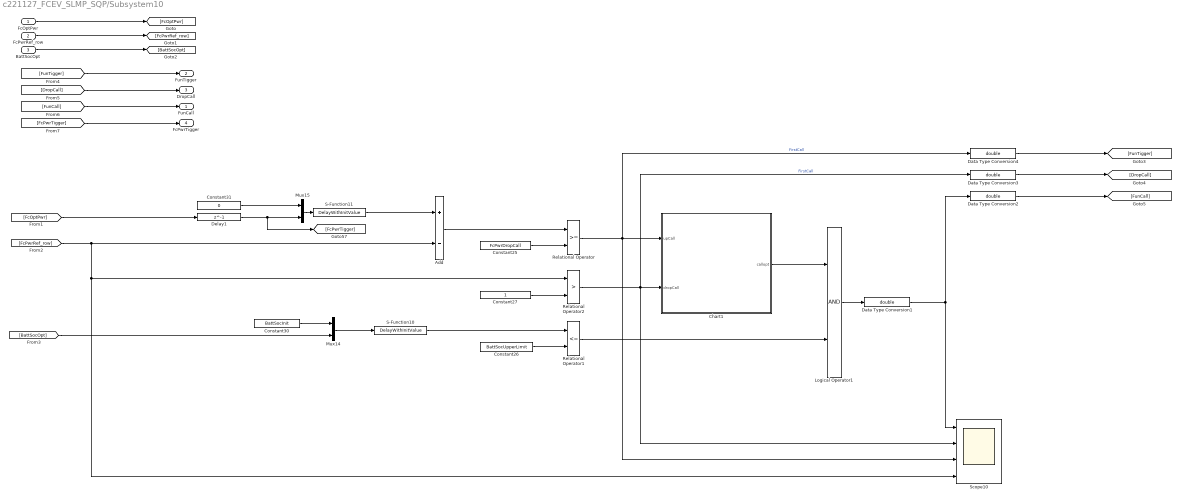
== system c221127_FCEV_SLMP_SQP/Subsystem10 ==
  FcOptPwr : Inport
  FcPwrRef_row : Inport  Port=2
  BattSocOpt : Inport  Port=3
  Add : Sum  Inputs=+-
  Chart1 : Stateflow chart  TreatAsAtomicUnit=on
  Constant25 : Constant  Value=FcPwrDropCall
  Constant26 : Constant  Value=BattSocUpperLimit
  Constant27 : Constant
  Constant30 : Constant  Value=BattSocInit
  Constant31 : Constant  Value=0
  Data Type Conversion{1..4} (4 alike) : DataTypeConversion  OutDataTypeStr=double  SaturateOnIntegerOverflow=off  RndMeth=Floor
  Delay1 : Delay  DelayLength=1
  Logical Operator1 : Logic
  Mux14 : Mux  Inputs=2
  Mux15 : Mux  Inputs=2
  Relational Operator : RelationalOperator
  Relational Operator1 : RelationalOperator  Operator=<=
  Relational Operator2 : RelationalOperator  Operator=>
  S-Function10 : S-Function  FunctionName=DelayWithInitValue  SFunctionDeploymentMode=off  EnableBusSupport=off
  S-Function11 : S-Function  FunctionName=DelayWithInitValue  SFunctionDeploymentMode=off  EnableBusSupport=off
  Scope10 : Scope  NumInputPorts=4
  FunCall : Outport
  FunTigger : Outport  Port=2
  DropCall : Outport  Port=3
  FcPwrTigger : Outport  Port=4
  wires:
  Constant30/1 -> Mux14/1
  Add/1 -> Relational Operator/1
  Chart1/1(callopt) -> Logical Operator1/1
  Logical Operator1/1 -> Data Type Conversion1/1
  Constant26/1 -> Relational Operator1/2
  Relational Operator2/1 -> Scope10/2, Data Type Conversion3/1, Chart1/2(dropCall)  "FirstCall"
  S-Function10/1 -> Relational Operator1/1
  Relational Operator/1 -> Scope10/3, Data Type Conversion4/1, Chart1/1(upCall)  "FirstCall"
  S-Function11/1 -> Add/1
  Constant31/1 -> Mux15/1
  Mux14/1 -> S-Function10/1
  Data Type Conversion1/1 -> Data Type Conversion2/1, Scope10/1
  Delay1/1 -> [FcPwrTigger], Mux15/2
  Mux15/1 -> S-Function11/1
  Constant27/1 -> Relational Operator2/2
  Relational Operator1/1 -> Logical Operator1/2
  Constant25/1 -> Relational Operator/2
  Data Type Conversion3/1 -> [DropCall]
  Data Type Conversion4/1 -> [FunTigger]
  [FcPwrRef_row] -> Relational Operator2/1, Scope10/4, Add/2
  [FcOptPwr] -> Delay1/1
  [BattSocOpt] -> Mux14/2
  Data Type Conversion2/1 -> [FunCall]
  FcOptPwr/1 -> [FcOptPwr]
  FcPwrRef_row/1 -> [FcPwrRef_row]
  BattSocOpt/1 -> [BattSocOpt]
  [FcPwrTigger] -> FcPwrTigger/1
  [FunCall] -> FunCall/1
  [DropCall] -> DropCall/1
  [FunTigger] -> FunTigger/1

== system c221127_FCEV_SLMP_SQP/Subsystem2 ==
  note: Thermal Model (Cell)
  note: Electrical Model
  BattReqPwrKw : Inport
  Add : Sum
  Capacity Degradation Model (Cell)1 : Subsystem
  Constant : Constant  Value=BattInitTemp
  Electrical Model1 : Subsystem  Tag=electrical
  Gain : Gain  Gain=0.5
  Gain1 : Gain  Gain=1000
  MATLAB Function1 : MATLAB Function  TreatAsAtomicUnit=on
  Mux : Mux  Inputs=2
  S-Function : S-Function  FunctionName=DelayWithInitValue  SFunctionDeploymentMode=off  EnableBusSupport=off
  Thermal Model1 : Subsystem
  BattSocOpt : Outport
  BattOpPwr : Outport  Port=2
  BattDegRmb : Outport  Port=3
  wires:
  [BattReqPwr_w] -> Electrical Model1/2(BattPwr_w)
  Electrical Model1/4(Pb,ava) -> [BattOpPwr]
  Thermal Model1/2(Ts.) -> [BattTemp_s]
  Electrical Model1/2(SOC) -> [BattSoc]
  Electrical Model1/3(I) -> [BattCurrent]
  [BattTemp] -> Mux/2
  [BattTemp] -> Capacity Degradation Model (Cell)1/1(Temp (oC))
  [BattCurrent] -> Capacity Degradation Model (Cell)1/3(I(A))
  [BattSoc] -> Capacity Degradation Model (Cell)1/2(SOC)
  Electrical Model1/1(Qb) -> [Batt_Qb]
  [Batt_Qb] -> Thermal Model1/1(Qb)
  Thermal Model1/1(Tc.) -> [BattTemp_c]
  [BattTemp_c] -> Add/2
  [BattTemp_s] -> Add/1
  Add/1 -> Gain/1
  Gain/1 -> [BattTemp]
  BattReqPwrKw/1 -> Gain1/1
  [BattSoc] -> BattSocOpt/1
  [BattOpPwr] -> BattOpPwr/1
  Gain1/1 -> [BattReqPwr_w]
  S-Function/1 -> Electrical Model1/1(BattTemp)
  Mux/1 -> S-Function/1
  Constant/1 -> Mux/1
  [BattOpPwr] -> MATLAB Function1/1(BattPwrKw)
  [BattSoc] -> MATLAB Function1/2(BattSocOpt)
  MATLAB Function1/1(BattDegRmb) -> [BattDegRmb]
  [BattDegRmb] -> BattDegRmb/1

== system c221127_FCEV_SLMP_SQP/Subsystem3 ==
  note: Direct Hydrogen PEM Fuel Cell
  note: Note: Speed NOT used; carried only for compatability.
  note: 不虑DC/DC转换器
  FC on : Inport
  "FC_pwr kW " : Inport  Port=2
  DC/DC efficiency : Lookup_n-D  NumberOfTableDimensions=1  BreakpointsForDimension1=DCDC_ori_power_kW  Table=DCDC_ori_eff  RndMeth=Simplest
  Divide2 : Product  Inputs=**
  FcDegCountingSubSys : Subsystem
  Fuel Rate Calculation1 : Subsystem
  Fuel cell efficiency calculation : Subsystem
  Gain : Gain  Gain=1/1000
  HydpriceRmb : Gain  Gain=HydpriceRmb
  Integrator : Integrator
  Power Calculation : Subsystem
  Saturation1 : Saturate  UpperLimit=FC_power_max_kW  LowerLimit=FC_power_min_kW
  Saturation2 : Saturate  UpperLimit=FC_power_max_kW  LowerLimit=FC_power_min_kW
  Scope : Scope  NumInputPorts=2
  Scope2 : Scope
  To Workspace1 : ToWorkspace  VariableName=Hyd_con_rmb  SampleTime=-1
  To Workspace5 : ToWorkspace  VariableName=FC_eff  SampleTime=-1
  To Workspace9 : ToWorkspace  VariableName=FC_power_kW  SampleTime=-1
  FC power output avaliable to bus (kW) : Outport
  FcDegMux : Outport  Port=2
  FcDegSum : Outport  Port=3
  FcDegTransient : Outport  Port=4
  HydConRmb : Outport  Port=5
  HydConRate : Outport  Port=6
  tag scope: FC_fuel_consume_kg=global, FC_fuel_rate_gps=global, FC_power_kW=global
  wires:
  Saturation2/1 -> FcDegCountingSubSys/1(P_fc), Fuel cell efficiency calculation/1(fc power)
  Divide2/1 -> FC power output avaliable to bus (kW)/1
  Fuel Rate Calculation1/1(fcv_H2_rate (g/s)1) -> Integrator/1, [FC_fuel_rate_gps]
  Fuel cell efficiency calculation/1("fc_eff ") -> To Workspace5/1
  Saturation1/1 -> DC/DC efficiency/1, Scope2/1, [FC_power_kW], To Workspace9/1, Divide2/2, Saturation2/1, Fuel Rate Calculation1/1(fc pwr)
  FcDegCountingSubSys/2(FcDegSum) -> FcDegSum/1
  FcDegCountingSubSys/1(FcDegMux) -> FcDegMux/1
  DC/DC efficiency/1 -> Divide2/1
  Gain/1 -> [FC_fuel_consume_kg]
  FC on/1 -> Power Calculation/1(fc on)
  Power Calculation/1(Power output (kW)) -> Saturation1/1
  "FC_pwr kW "/1 -> Power Calculation/2(Power command (kW))
  Integrator/1 -> Gain/1
  FcDegCountingSubSys/3(FcDegTransient) -> FcDegTransient/1
  [FC_fuel_consume_kg] -> HydpriceRmb/1
  [FC_fuel_rate_gps] -> Scope/2
  [FC_fuel_consume_kg] -> Scope/1
  HydpriceRmb/1 -> To Workspace1/1, HydConRmb/1
  [FC_fuel_rate_gps] -> HydConRate/1

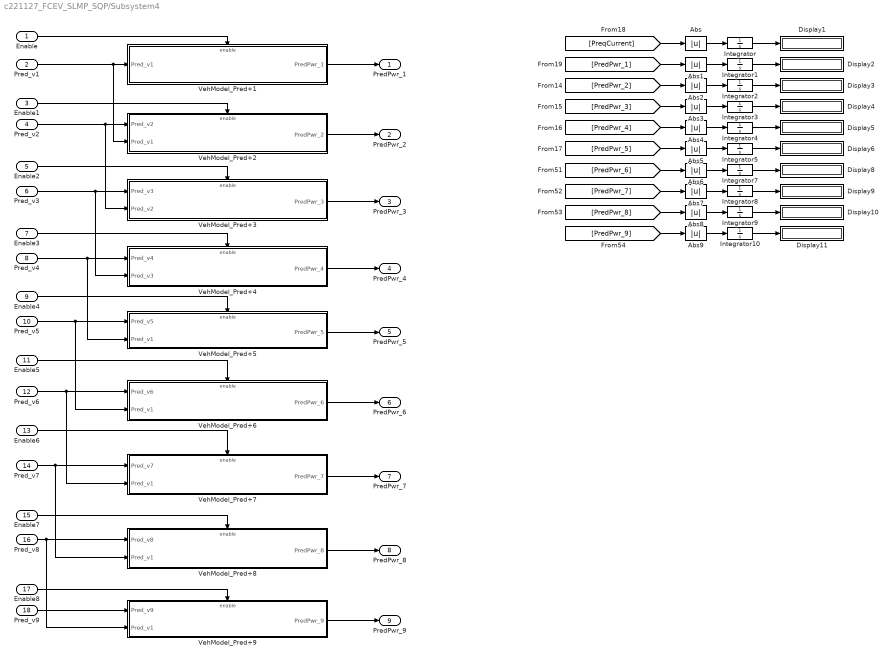
== system c221127_FCEV_SLMP_SQP/Subsystem4 ==
  Enable : Inport
  Pred_v1 : Inport  Port=2
  Enable1 : Inport  Port=3
  Pred_v2 : Inport  Port=4
  Enable2 : Inport  Port=5
  Pred_v3 : Inport  Port=6
  Enable3 : Inport  Port=7
  Pred_v4 : Inport  Port=8
  Enable4 : Inport  Port=9
  Pred_v5 : Inport  Port=10
  Enable5 : Inport  Port=11
  Pred_v6 : Inport  Port=12
  Enable6 : Inport  Port=13
  Pred_v7 : Inport  Port=14
  Enable7 : Inport  Port=15
  Pred_v8 : Inport  Port=16
  Enable8 : Inport  Port=17
  Pred_v9 : Inport  Port=18
  Abs{,1..9} (10 alike) : Abs  SaturateOnIntegerOverflow=off
  Display{1..6,8..11} (10 alike) : Display
  Integrator{,1..5,7..10} (10 alike) : Integrator
  VehModel_Pred+1 : Subsystem
  VehModel_Pred+2 : Subsystem
  VehModel_Pred+3 : Subsystem
  VehModel_Pred+4 : Subsystem
  VehModel_Pred+5 : Subsystem
  VehModel_Pred+6 : Subsystem
  VehModel_Pred+7 : Subsystem
  VehModel_Pred+8 : Subsystem
  VehModel_Pred+9 : Subsystem
  PredPwr_1 : Outport
  PredPwr_2 : Outport  Port=2
  PredPwr_3 : Outport  Port=3
  PredPwr_4 : Outport  Port=4
  PredPwr_5 : Outport  Port=5
  PredPwr_6 : Outport  Port=6
  PredPwr_7 : Outport  Port=7
  PredPwr_8 : Outport  Port=8
  PredPwr_9 : Outport  Port=9
  wires:
  Pred_v1/1 -> VehModel_Pred+2/2(Pred_v1), VehModel_Pred+1/1(Pred_v1)
  Pred_v3/1 -> VehModel_Pred+4/2(Pred_v3), VehModel_Pred+3/1(Pred_v3)
  Enable7/1 -> VehModel_Pred+8/Enable
  Enable6/1 -> VehModel_Pred+7/Enable
  VehModel_Pred+1/1(PredPwr_1) -> PredPwr_1/1
  Enable8/1 -> VehModel_Pred+9/Enable
  VehModel_Pred+7/1(PredPwr_7) -> PredPwr_7/1
  Enable1/1 -> VehModel_Pred+2/Enable
  VehModel_Pred+6/1(PredPwr_6) -> PredPwr_6/1
  Enable5/1 -> VehModel_Pred+6/Enable
  VehModel_Pred+9/1(PredPwr_9) -> PredPwr_9/1
  VehModel_Pred+3/1(PredPwr_3) -> PredPwr_3/1
  Pred_v9/1 -> VehModel_Pred+9/1(Pred_v9)
  Enable/1 -> VehModel_Pred+1/Enable
  Pred_v5/1 -> VehModel_Pred+6/2(Pred_v1), VehModel_Pred+5/1(Pred_v5)
  Pred_v2/1 -> VehModel_Pred+3/2(Pred_v2), VehModel_Pred+2/1(Pred_v2)
  VehModel_Pred+5/1(PredPwr_5) -> PredPwr_5/1
  VehModel_Pred+4/1(PredPwr_4) -> PredPwr_4/1
  Pred_v7/1 -> VehModel_Pred+7/1(Pred_v7), VehModel_Pred+8/2(Pred_v1)
  Enable3/1 -> VehModel_Pred+4/Enable
  VehModel_Pred+2/1(PredPwr_2) -> PredPwr_2/1
  Pred_v4/1 -> VehModel_Pred+5/2(Pred_v1), VehModel_Pred+4/1(Pred_v4)
  Pred_v8/1 -> VehModel_Pred+8/1(Pred_v8), VehModel_Pred+9/2(Pred_v1)
  VehModel_Pred+8/1(PredPwr_8) -> PredPwr_8/1
  Pred_v6/1 -> VehModel_Pred+7/2(Pred_v1), VehModel_Pred+6/1(Pred_v6)
  Enable4/1 -> VehModel_Pred+5/Enable
  Enable2/1 -> VehModel_Pred+3/Enable
  Integrator8/1 -> Display9/1
  Integrator2/1 -> Display3/1
  Integrator5/1 -> Display6/1
  Abs2/1 -> Integrator2/1
  Integrator3/1 -> Display4/1
  [PredPwr_5] -> Abs5/1
  [PredPwr_4] -> Abs4/1
  [PredPwr_2] -> Abs2/1
  Integrator1/1 -> Display2/1
  [PredPwr_1] -> Abs1/1
  Abs7/1 -> Integrator8/1
  [PredPwr_3] -> Abs3/1
  Abs5/1 -> Integrator5/1
  [PredPwr_9] -> Abs9/1
  Integrator4/1 -> Display5/1
  Integrator/1 -> Display1/1
  Abs1/1 -> Integrator1/1
  Abs6/1 -> Integrator7/1
  Integrator7/1 -> Display8/1
  [PredPwr_6] -> Abs6/1
  [PredPwr_7] -> Abs7/1
  Abs/1 -> Integrator/1
  Abs8/1 -> Integrator9/1
  [PreqCurrent] -> Abs/1
  Integrator10/1 -> Display11/1
  [PredPwr_8] -> Abs8/1
  Abs4/1 -> Integrator4/1
  Abs3/1 -> Integrator3/1
  Integrator9/1 -> Display10/1
  Abs9/1 -> Integrator10/1

== system c221127_FCEV_SLMP_SQP/Subsystem5 ==
  In1 : Inport
  In3 : Inport  Port=2
  In4 : Inport  Port=3
  In5 : Inport  Port=4
  In2 : Inport  Port=5
  In6 : Inport  Port=6
  Demux2 : Demux  Outputs=3
  Mux4 : Mux  Inputs=2
  To Workspace1 : ToWorkspace  VariableName=DegSum  SampleTime=-1
  To Workspace15 : ToWorkspace  VariableName=FcOptPwrComp  SampleTime=-1
  To Workspace2 : ToWorkspace  VariableName=HighPwrDeg  SampleTime=-1
  To Workspace3 : ToWorkspace  VariableName=LowPwrDeg  SampleTime=-1
  To Workspace4 : ToWorkspace  VariableName=PwrShiftDeg  SampleTime=-1
  To Workspace5 : ToWorkspace  VariableName=FcDegTransient  SampleTime=-1
  To Workspace6 : ToWorkspace  VariableName=HydConRmbIst  SampleTime=-1
  FcOptPwrComp : Outport
  PwrShiftDeg : Outport  Port=2
  FcDegTransient : Outport  Port=3
  HydConRmbIst : Outport  Port=4
  LowPwrDeg : Outport  Port=5
  HighPwrDeg : Outport  Port=6
  DegSum : Outport  Port=7
  wires:
  Mux4/1 -> FcOptPwrComp/1, To Workspace15/1
  Demux2/2 -> To Workspace3/1, LowPwrDeg/1  "LowPwrDeg"
  Demux2/3 -> To Workspace4/1, PwrShiftDeg/1  "PwrShiftDeg"
  Demux2/1 -> To Workspace2/1, HighPwrDeg/1  "HighPwrDeg"
  In4/1 -> To Workspace1/1, DegSum/1  "FcDegSum"
  In3/1 -> Mux4/2  "Ref"
  In1/1 -> Mux4/1  "Opt"
  In5/1 -> Demux2/1
  In2/1 -> To Workspace5/1, FcDegTransient/1
  In6/1 -> To Workspace6/1, HydConRmbIst/1

== system c221127_FCEV_SLMP_SQP/Subsystem6 ==
  In1 : Inport
  In2 : Inport  Port=2
  In3 : Inport  Port=3
  Add : Sum
  Mux5 : Mux  Inputs=2
  FcPwrRef : Outport
  BattPwrRef : Outport  Port=2
  CprWithPreq : Outport  Port=3
  wires:
  In1/1 -> FcPwrRef/1, Add/1
  In3/1 -> Mux5/2
  Add/1 -> Mux5/1
  Mux5/1 -> CprWithPreq/1
  In2/1 -> BattPwrRef/1, Add/2

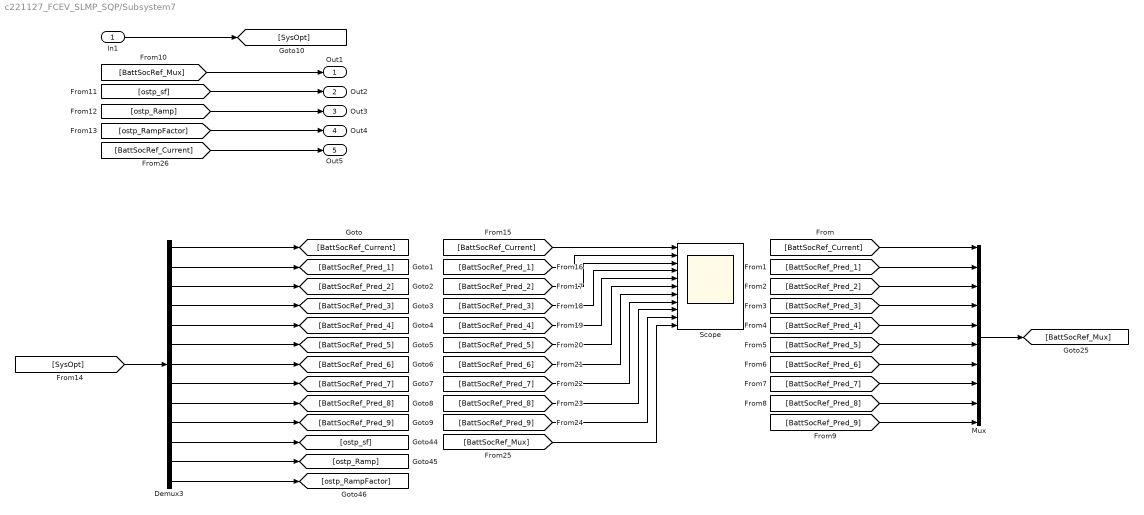
== system c221127_FCEV_SLMP_SQP/Subsystem7 ==
  In1 : Inport
  Demux3 : Demux  Outputs=13
  Mux : Mux  Inputs=10
  Scope : Scope  NumInputPorts=11
  Out1 : Outport
  Out2 : Outport  Port=2
  Out3 : Outport  Port=3
  Out4 : Outport  Port=4
  Out5 : Outport  Port=5
  wires:
  Demux3/5 -> [BattSocRef_Pred_4]
  Demux3/10 -> [BattSocRef_Pred_9]
  Demux3/6 -> [BattSocRef_Pred_5]
  Demux3/1 -> [BattSocRef_Current]
  Demux3/2 -> [BattSocRef_Pred_1]
  Demux3/3 -> [BattSocRef_Pred_2]
  Demux3/4 -> [BattSocRef_Pred_3]
  Demux3/7 -> [BattSocRef_Pred_6]
  Demux3/9 -> [BattSocRef_Pred_8]
  Demux3/8 -> [BattSocRef_Pred_7]
  Demux3/11 -> [ostp_sf]
  Demux3/12 -> [ostp_Ramp]
  Demux3/13 -> [ostp_RampFactor]
  [BattSocRef_Pred_9] -> Mux/10
  [BattSocRef_Pred_8] -> Mux/9
  [BattSocRef_Pred_7] -> Mux/8
  [BattSocRef_Pred_6] -> Mux/7
  [BattSocRef_Pred_5] -> Mux/6
  [BattSocRef_Pred_4] -> Mux/5
  [BattSocRef_Pred_3] -> Mux/4
  [BattSocRef_Pred_2] -> Mux/3
  [BattSocRef_Pred_1] -> Mux/2
  [BattSocRef_Current] -> Mux/1
  Mux/1 -> [BattSocRef_Mux]
  [BattSocRef_Mux] -> Out1/1
  [ostp_sf] -> Out2/1
  [ostp_Ramp] -> Out3/1
  [ostp_RampFactor] -> Out4/1
  In1/1 -> [SysOpt]
  [SysOpt] -> Demux3/1
  [BattSocRef_Current] -> Scope/1
  [BattSocRef_Pred_1] -> Scope/2
  [BattSocRef_Pred_2] -> Scope/3
  [BattSocRef_Pred_3] -> Scope/4
  [BattSocRef_Pred_4] -> Scope/5
  [BattSocRef_Pred_5] -> Scope/6
  [BattSocRef_Pred_6] -> Scope/7
  [BattSocRef_Pred_7] -> Scope/8
  [BattSocRef_Pred_8] -> Scope/9
  [BattSocRef_Pred_9] -> Scope/10
  [BattSocRef_Mux] -> Scope/11
  [BattSocRef_Current] -> Out5/1

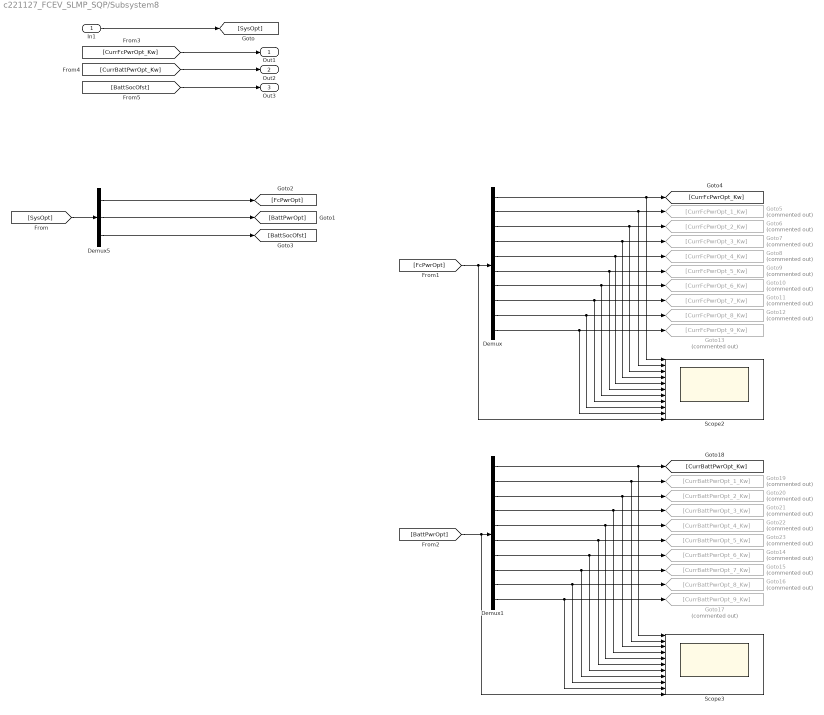
== system c221127_FCEV_SLMP_SQP/Subsystem8 ==
  In1 : Inport
  Demux : Demux  Outputs=10
  Demux1 : Demux  Outputs=10
  Demux5 : Demux  Outputs=3
  Goto10 : Goto  Commented=on  GotoTag=CurrFcPwrOpt_6_Kw
  Goto11 : Goto  Commented=on  GotoTag=CurrFcPwrOpt_7_Kw
  Goto12 : Goto  Commented=on  GotoTag=CurrFcPwrOpt_8_Kw
  Goto13 : Goto  Commented=on  GotoTag=CurrFcPwrOpt_9_Kw
  Goto14 : Goto  Commented=on  GotoTag=CurrBattPwrOpt_6_Kw
  Goto15 : Goto  Commented=on  GotoTag=CurrBattPwrOpt_7_Kw
  Goto16 : Goto  Commented=on  GotoTag=CurrBattPwrOpt_8_Kw
  Goto17 : Goto  Commented=on  GotoTag=CurrBattPwrOpt_9_Kw
  Goto19 : Goto  Commented=on  GotoTag=CurrBattPwrOpt_1_Kw
  Goto20 : Goto  Commented=on  GotoTag=CurrBattPwrOpt_2_Kw
  Goto21 : Goto  Commented=on  GotoTag=CurrBattPwrOpt_3_Kw
  Goto22 : Goto  Commented=on  GotoTag=CurrBattPwrOpt_4_Kw
  Goto23 : Goto  Commented=on  GotoTag=CurrBattPwrOpt_5_Kw
  Goto5 : Goto  Commented=on  GotoTag=CurrFcPwrOpt_1_Kw
  Goto6 : Goto  Commented=on  GotoTag=CurrFcPwrOpt_2_Kw
  Goto7 : Goto  Commented=on  GotoTag=CurrFcPwrOpt_3_Kw
  Goto8 : Goto  Commented=on  GotoTag=CurrFcPwrOpt_4_Kw
  Goto9 : Goto  Commented=on  GotoTag=CurrFcPwrOpt_5_Kw
  Scope2 : Scope  NumInputPorts=11
  Scope3 : Scope  NumInputPorts=11
  Out1 : Outport
  Out2 : Outport  Port=2
  Out3 : Outport  Port=3
  wires:
  Demux5/2 -> [BattPwrOpt]
  [SysOpt] -> Demux5/1
  Demux5/1 -> [FcPwrOpt]
  Demux5/3 -> [BattSocOfst]
  In1/1 -> [SysOpt]
  [FcPwrOpt] -> Scope2/11, Demux/1
  Demux/1 -> Scope2/1, [CurrFcPwrOpt_Kw]
  Demux/2 -> Scope2/2, Goto5/1
  Demux/3 -> Scope2/3, Goto6/1
  Demux/4 -> Scope2/4, Goto7/1
  Demux/5 -> Scope2/5, Goto8/1
  Demux/6 -> Scope2/6, Goto9/1
  Demux/7 -> Scope2/7, Goto10/1
  Demux/8 -> Scope2/8, Goto11/1
  Demux/9 -> Scope2/9, Goto12/1
  Demux/10 -> Scope2/10, Goto13/1
  Demux1/10 -> Scope3/10, Goto17/1
  Demux1/9 -> Scope3/9, Goto16/1
  Demux1/8 -> Scope3/8, Goto15/1
  Demux1/7 -> Scope3/7, Goto14/1
  Demux1/6 -> Scope3/6, Goto23/1
  Demux1/5 -> Scope3/5, Goto22/1
  Demux1/4 -> Scope3/4, Goto21/1
  Demux1/3 -> Scope3/3, Goto20/1
  Demux1/2 -> Scope3/2, Goto19/1
  Demux1/1 -> Scope3/1, [CurrBattPwrOpt_Kw]
  [BattPwrOpt] -> Scope3/11, Demux1/1
  [CurrFcPwrOpt_Kw] -> Out1/1
  [CurrBattPwrOpt_Kw] -> Out2/1
  [BattSocOfst] -> Out3/1

== system c221127_FCEV_SLMP_SQP/SuperCapacitor ==
  P : Inport
  In2 : Inport  Port=2
  Add1 : Sum  Inputs=+-
  Clock1 : Clock
  Constant10 : Constant  Value=20
  Constant11 : Constant  Value=0
  Constant12 : Constant
  Constant13 : Constant  Value=2.4
  Constant14 : Constant  Value=SC_iv
  Constant15 : Constant  Value=SC_rc
  Constant2 : Constant  Value=SC_nm*SC_np*SC_ns
  Constant3 : Constant  Value=6000
  Display2 : Display
  MATLAB Function1 : MATLAB Function  TreatAsAtomicUnit=on
  Manual Switch2 : ManualSwitch  CurrentSetting=0
  Manual Switch3 : ManualSwitch
  Memory1 : Memory
  SC_Volt_2_Soc1 : Lookup_n-D  NumberOfTableDimensions=1  BreakpointsForDimension1=SC_SocTable(:,1)  Table=SC_SocTable(:,2)  InternalRulePriority=Speed  RndMeth=Simplest
  Scope1 : Scope  NumInputPorts=3
  Stop Simulation1 : Stop
  Switch2 : Switch  Criteria=u2 > Threshold  Threshold=1  SaturateOnIntegerOverflow=off  InputSameDT=off
  Switch3 : Switch  Criteria=u2 > Threshold  SaturateOnIntegerOverflow=off  InputSameDT=off
  Out1 : Outport
  wires:
  Switch3/1 -> Stop Simulation1/1
  Constant12/1 -> Switch3/3
  Constant10/1 -> Add1/2
  SC_Volt_2_Soc1/1 -> [SC_soc], Scope1/1, Add1/1
  Constant3/1 -> Manual Switch3/2
  P/1 -> [PwrInput]
  Clock1/1 -> Switch2/2, Display2/1
  MATLAB Function1/1(y) -> SC_Volt_2_Soc1/1, Scope1/2, Memory1/1
  Add1/1 -> Switch3/2
  Constant15/1 -> Manual Switch3/1
  Constant14/1 -> Manual Switch2/1
  Constant11/1 -> Switch3/1
  Constant2/1 -> MATLAB Function1/2(n)
  Manual Switch2/1 -> Switch2/3
  Constant13/1 -> Manual Switch2/2
  Memory1/1 -> Switch2/1
  Switch2/1 -> MATLAB Function1/4(u_k)
  Manual Switch3/1 -> MATLAB Function1/3(c)
  In2/1 -> Scope1/3
  [PwrInput] -> MATLAB Function1/1(P)
  [SC_soc] -> Out1/1

== system c221127_FCEV_SLMP_SQP/VehModel_Current ==
  note: CarryOver
  Vcurrent : Inport
  BattPwrKw : Inport  Port=2
  FcPwrKw : Inport  Port=3
  Delay : Delay  DelayLength=1
  Delay1 : Delay  DelayLength=1
  Gain : Gain  Gain=3.6
  Power bus : Subsystem
  主减及变速器模型 : Subsystem
  整车动力学模型 : Subsystem
  车轮模型 : Subsystem
  驱动电机模型 : Subsystem
  PreqCurrent : Outport
  wires:
  主减及变速器模型/1(drive torque (Nm) speed (rad/s) brike torque (Nm) req'd at input side of final drive) -> 驱动电机模型/1(drive torque (Nm) speed (rad/s) brake torque (Nm) req'd at motor)
  驱动电机模型/1(drive power (kW) brake power (kW) req'd motor input power (电功率)) -> Power bus/1(drive power (kW) brake power (kW) req at power bus)
  驱动电机模型/2(drive torque (Nm) brake torque (Nm) speed avail (rad/s) avail. at rotor) -> 主减及变速器模型/2(drive torque (Nm) brake torque (Nm) speed avail (rad/s) at input side of final drive)
  主减及变速器模型/2(drive torque (Nm) brake torque (Nm) speed avail (rad/s) at output side of final drive) -> 车轮模型/2("drive torque (Nm) brake torque (Nm) speed (rad/s) available from drivetrain into axle ")
  车轮模型/2(tractive force (N) brake force (N) linear speed achievable (m/s)) -> 整车动力学模型/2(实际车辆驱动力N 制动力N 和车速m/s)
  整车动力学模型/1(需求驱动力N 目标车速m/s 需求制动力N) -> 车轮模型/1("tractive force, brake force and speed req'd of tire/road interface 需求驱动力N 目标车速m/s 需求制动力N")
  车轮模型/1(drive torque (Nm) speed (rad/s) brake torque (Nm) req'd from drivetrain into axle) -> 主减及变速器模型/1(drive torque (Nm) speed (rad/s) brake torque (Nm) req'd at output side of final drive)
  Vcurrent/1 -> Gain/1
  Power bus/2(drive power (kW) brake power (kW) availableat power bus) -> 驱动电机模型/2(drive power (kW) brake power (kW) input available motor)
  Power bus/1(drive power (kW)/brake power (kW) req from power sources) -> [PreqCurrent]
  Gain/1 -> [Vcurrent_kph]
  Delay/1 -> Power bus/2(pwr availible from battery kW)
  Delay1/1 -> Power bus/3(pwr availible from FC_+DCDC kW)
  [Vcurrent_kph] -> 整车动力学模型/1(需求车速 km/h)
  [BattPwr_kw] -> Delay/1
  [FcPwr_kw] -> Delay1/1
  BattPwrKw/1 -> [BattPwr_kw]
  FcPwrKw/1 -> [FcPwr_kw]
  [PreqCurrent] -> PreqCurrent/1
